simulink model "PenduloSimulink"  (R2025b)
settings: Solver=VariableStepAuto  StartTime=0.0  StopTime=10.0  RelTol=1e-3
undefined symbols (not defined in the file): Beq, Bp, g, Ip, lp, Mc, Mp
settings Model: Creator=Cecilia  LastModifiedBy=Cecilia

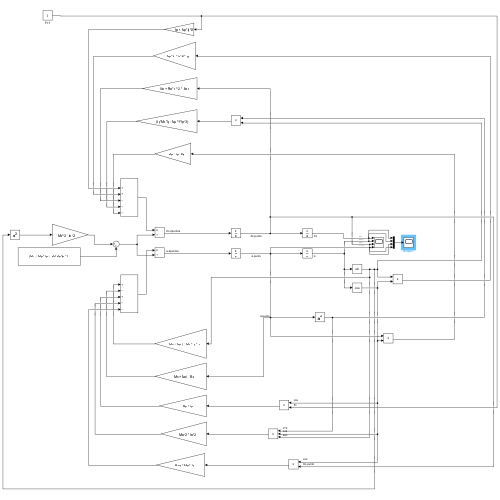
[thumbnail: Simulink's stored preview of the top-level diagram]
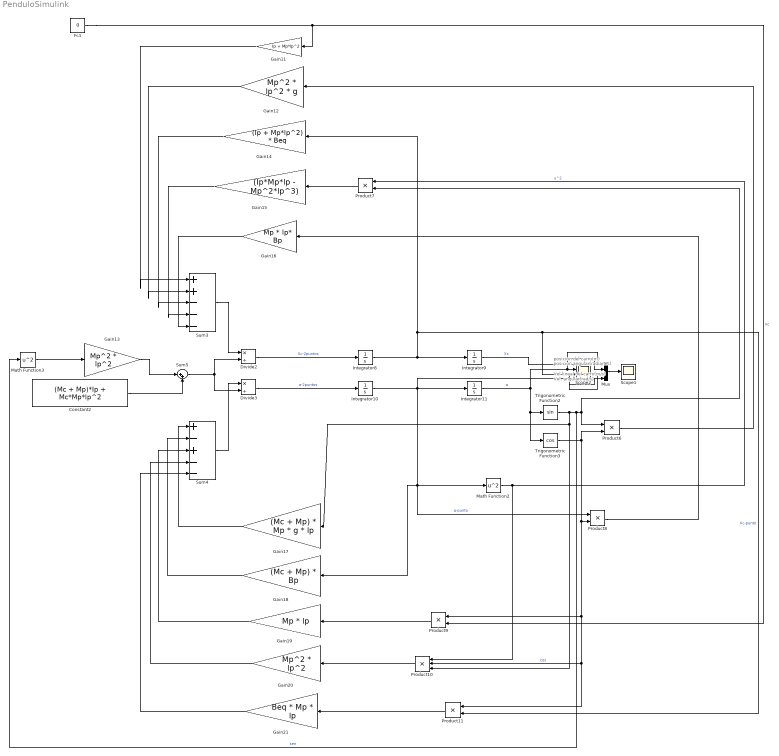
== system PenduloSimulink ==
  note: posicion del carro(m)
  note: Vel lineal del carro(m/s)
  note: posicion angular(radianes)
  note: Vel. angular(rad/s)
  Constant2 : Constant  Value=(Mc + Mp)*Ip + Mc*Mp*lp^2
  Divide2 : Product  Inputs=*/
  Divide3 : Product  Inputs=*/
  Fc1 : Constant  Value=0
  Gain11 : Gain  Gain=Ip + Mp*lp^2
  Gain12 : Gain  Gain=Mp^2 * lp^2 * g
  Gain13 : Gain  Gain=Mp^2 * lp^2
  Gain14 : Gain  Gain=(Ip + Mp*lp^2) * Beq
  Gain15 : Gain  Gain=(Ip*Mp*lp - Mp^2*lp^3)
  Gain16 : Gain  Gain=Mp * lp* Bp
  Gain17 : Gain  Gain=(Mc + Mp) * Mp * g * lp
  Gain18 : Gain  Gain=(Mc + Mp) * Bp
  Gain19 : Gain  Gain=Mp * lp
  Gain20 : Gain  Gain=Mp^2 * lp^2
  Gain21 : Gain  Gain=Beq * Mp * lp
  Integrator10 : Integrator
  Integrator11 : Integrator  InitialCondition=1*(pi/180)
  Integrator8 : Integrator
  Integrator9 : Integrator
  Math Function2 : Math  Operator=square
  Math Function3 : Math  Operator=square
  Mux : Mux
  Product10 : Product  Inputs=3
  Product{6..9,11} (5 alike) : Product
  Scope1 : Scope
      settings: ActiveDisplayYMinimum=-13.187671205503406  ActiveDisplayYMaximum=110.94267267436797
  Scope2 : Scope  NumInputPorts=4
      settings: ActiveDisplayYMinimum=-0.02865830537247703  ActiveDisplayYMaximum=0.21765477317458878  DataLoggingVariableName=ScopeData2
  Sum3 : Sum  Inputs=|++---
  Sum4 : Sum  Inputs=|+-+--
  Sum5 : Sum  Inputs=|++
  Trigonometric Function2 : Trigonometry
  Trigonometric Function3 : Trigonometry  Operator=cos
  wires:
  Gain14/1 -> Sum3/3
  Integrator11/1 -> Trigonometric Function3/1, Trigonometric Function2/1, Scope2/2, Mux/2  "α"
  Sum4/1 -> Divide3/1
  Gain17/1 -> Sum4/1
  Gain13/1 -> Sum5/1
  Constant2/1 -> Sum5/2
  Product9/1 -> Gain19/1
  Product11/1 -> Gain21/1
  Integrator8/1 -> Product11/2, Scope2/3, Mux/3, Gain14/1, Integrator9/1  "Xc-punto"
  Product8/1 -> Gain16/1
  Integrator9/1 -> Scope2/1, Mux/1  "Xc"
  Gain19/1 -> Sum4/3
  Gain12/1 -> Sum3/2
  Math Function3/1 -> Gain13/1
  Mux/1 -> Scope1/1
  Trigonometric Function3/1 -> Product11/1, Product10/2, Product9/1, Product8/2, Product6/2  "cos"
  Gain20/1 -> Sum4/4
  Sum5/1 -> Divide3/2, Divide2/2
  Gain11/1 -> Sum3/1
  Product6/1 -> Gain12/1
  Gain16/1 -> Sum3/5
  Sum3/1 -> Divide2/1
  Divide3/1 -> Integrator10/1  "α-2puntos"
  Math Function2/1 -> Product10/1, Product7/1  "u^2"
  Gain18/1 -> Sum4/2
  Product10/1 -> Gain20/1
  Integrator10/1 -> Product8/1, Gain18/1, Math Function2/1, Scope2/4, Mux/4, Integrator11/1  "α-punto"
  Gain15/1 -> Sum3/4
  Product7/1 -> Gain15/1
  Fc1/1 -> Product9/2, Gain11/1  "Fc"
  Divide2/1 -> Integrator8/1  "Xc-2puntos"
  Trigonometric Function2/1 -> Math Function3/1, Product6/1, Product7/2, Product10/3, Gain17/1  "sen"
  Gain21/1 -> Sum4/5
